simulink model "EKF_LQR_PID"  (R2024b)
settings: Solver=VariableStepAuto  StartTime=0.0  StopTime=10  FixedStep=0.001  RelTol=1e-3
values from neighbouring files (symbols this model uses):
  A = [0 1 0 0 0 0 ... (first row only)    [main.m]
  B = [0;1/mc;0;-1/mb;0;-1/(l*mc)]    [main.m]
  C = [1 0 0 0 l 0]    [main.m]
  dT = param.Ts    [main.m]
  Kd = 0.8    [main.m]
  Ki = 10    [main.m]
  Kp = 12    [main.m]
  l = 0.25    [main.m]
  L_gain = lqr(A,B,Q_LQR,R_LQR)    [main.m]
  LD = acker(system_l.A',system_l.C',poles)    [main.m]
  system_l = ss(A,B,C,D)    [main.m]
undefined symbols (not defined in the file or in its folder): denum, num, param
libraries: simulink x6, simulink_extras x6, slpidlib x1
settings Model: Creator=hospm  LastModifiedBy=elias

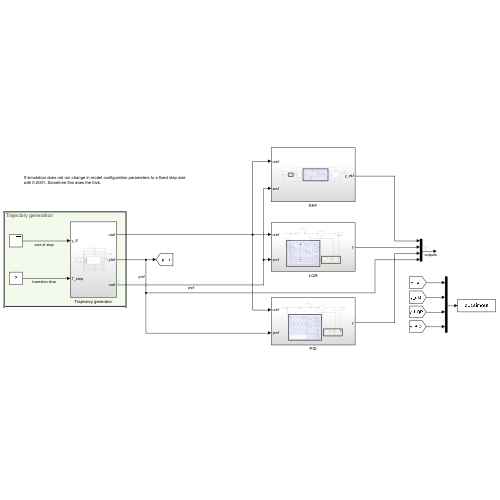
[thumbnail: Simulink's stored preview of the top-level diagram]
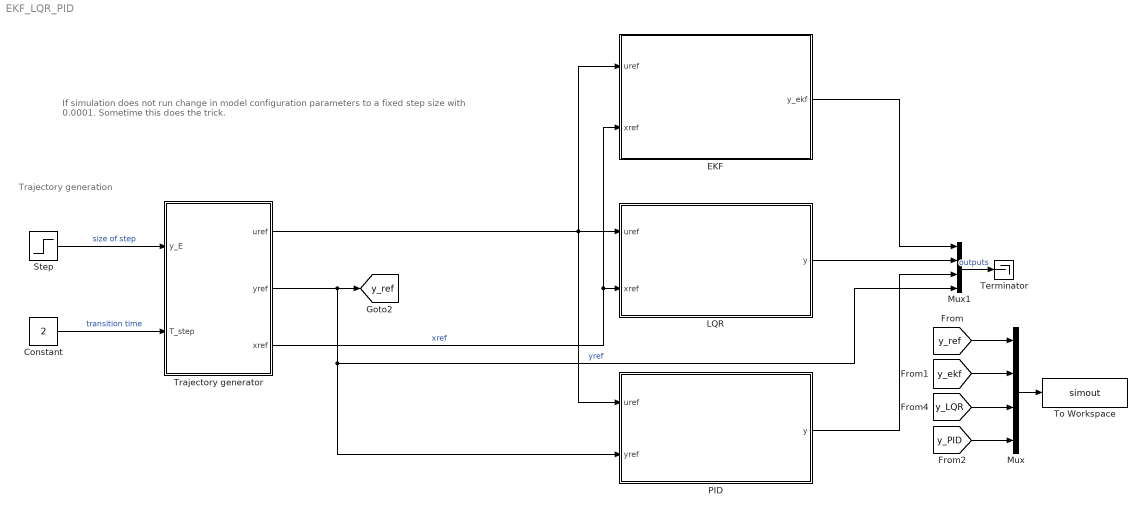
== system EKF_LQR_PID ==
  note: If simulation does not run change in model configuration parameters to a fixed step size with 0.0001. Sometime this does the trick.
  note: Trajectory generation
  Constant : Constant  Value=2
  EKF : Subsystem
  LQR : Subsystem
  Mux : Mux
  Mux1 : Mux
  PID : Subsystem
  Step : Step  Time=0  After=2  SampleTime=0
  Terminator : Terminator
  To Workspace : ToWorkspace  VariableName=simout  SaveFormat=Timeseries  SampleTime=-1
  Trajectory generator : Subsystem
  tag scope: y_ref=global
  wires:
  Constant/1 -> Trajectory generator/2(T_step)  "transition time"
  Trajectory generator/2(yref) -> Mux1/4, PID/2(yref), [y_ref]  "yref"
  Step/1 -> Trajectory generator/1(y_E)  "size of step"
  Mux/1 -> To Workspace/1
  [y_ref] -> Mux/1
  Trajectory generator/1(uref) -> PID/1(uref), EKF/1(uref), LQR/1(uref)
  Trajectory generator/3(xref) -> EKF/2(xref), LQR/2(xref)  "xref"
  EKF/1(y_ekf) -> Mux1/1
  Mux1/1 -> Terminator/1  "outputs"
  LQR/1(y) -> Mux1/2
  PID/1(y) -> Mux1/3
  [y_PID] -> Mux/4
  [y_LQR] -> Mux/3
  [y_ekf] -> Mux/2

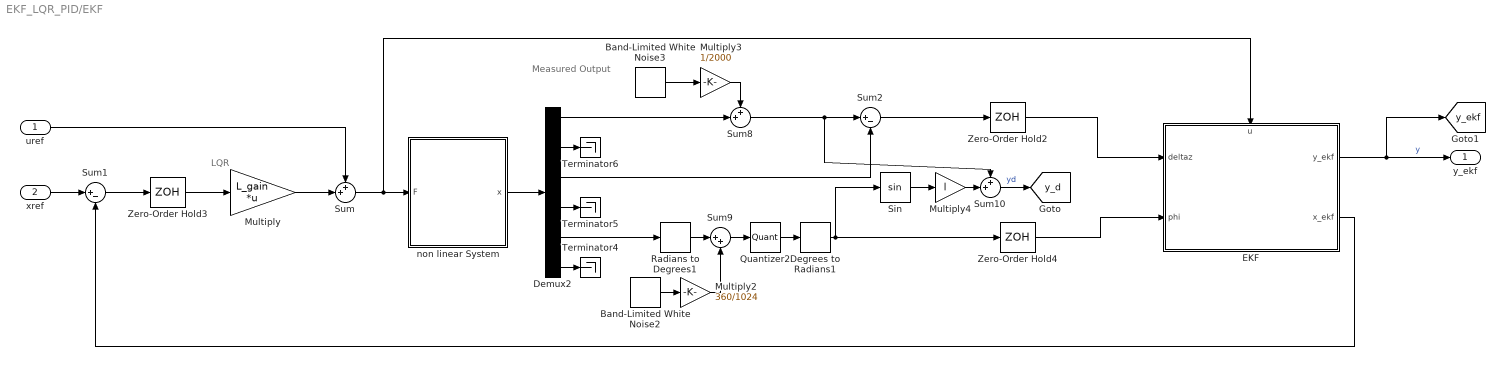
== system EKF_LQR_PID/EKF ==
  note: LQR
  note: Measured Output
  uref : Inport
  xref : Inport  Port=2
  Band-Limited White Noise2 : simulink/Sources/Band-Limited White Noise  Cov=[0.1]  Ts=0.1  seed=[23341]
  Band-Limited White Noise3 : simulink/Sources/Band-Limited White Noise  Cov=[0.1]  Ts=0.1  seed=[23341]
  Degrees to Radians1 : simulink_extras/Transformations/Degrees to Radians
  Demux2 : Demux  Outputs=6
  EKF : Subsystem
      settings: PortSchema="{\"entries\":[{\"content\":{\"sides\":[{\"content\":{\"connectorIds\":[\"In1\",\"In2\"]},\"type\":\"ConnectorPlacement.EquallySpacedRectSide\",\"uuid\":\"7d448900-18ad-41d5-8be7-5b2f8237e026\"},{\"content\":{\"connectorIds\":[\"Out1\",\"Out2\"],\"side\":\"RIGHT\"},\"type\":\"ConnectorPlacement.EquallySpacedRectSide\",\"uuid\":\"f5f89615-8db2-446f-9ddf-3fbf985b739e\"},{\"content\":{\"connectorIds\":[\"In3\"],\"side\":\"TOP\"},\"type\":\"ConnectorPlacement.EquallySpacedRectSide\",\"uuid\":\"59db8e0c-78e3-492a-b009-e31c80c69e55\"}]},\"type\":\"ConnectorPlacement.EquallySpacedConnector\",\"uuid\":\"488a84d0-998b-49ab-9f38-67f2321ad282\"}],\"packageUris\":[\"http://schema.mathworks.com/mf0/Connector/R2020b\"],\"version\":\"1.0\"}"
  Multiply : Gain  Gain=L_gain  Multiplication=Matrix(K*u) (u vector)
  Multiply2 : Gain  Gain=360/1024
  Multiply3 : Gain  Gain=1/2000
  Multiply4 : Gain  Gain=l
  Quantizer2 : Quantizer  QuantizationInterval=360/1024
  Radians to Degrees1 : simulink_extras/Transformations/Radians to Degrees
  Sin : Trigonometry
  Sum : Sum  Inputs=++|
  Sum1 : Sum  Inputs=|+-
  Sum10 : Sum  Inputs=++|
  Sum2 : Sum  Inputs=|+-
  Sum8 : Sum  Inputs=++|
  Sum9 : Sum  Inputs=|++
  Terminator4 : Terminator
  Terminator5 : Terminator
  Terminator6 : Terminator
  Zero-Order Hold2 : ZeroOrderHold  SampleTime=param.Ts
  Zero-Order Hold3 : ZeroOrderHold  SampleTime=param.Ts
  Zero-Order Hold4 : ZeroOrderHold  SampleTime=param.Ts
  non linear System : Subsystem
  y_ekf : Outport
  tag scope: y_d=global, y_ekf=global
  wires:
  Demux2/3 -> Sum2/2
  Multiply/1 -> Sum/2
  Degrees to Radians1/1 -> Sin/1, Zero-Order Hold4/1
  Sum9/1 -> Quantizer2/1
  Band-Limited White Noise3/1 -> Multiply3/1
  Zero-Order Hold3/1 -> Multiply/1
  EKF/2(x_ekf) -> Sum1/2
  Demux2/2 -> Terminator6/1
  Sum8/1 -> Sum2/1, Sum10/1
  Demux2/5 -> Radians to Degrees1/1
  Radians to Degrees1/1 -> Sum9/1
  Demux2/6 -> Terminator4/1
  Demux2/4 -> Terminator5/1
  Sum2/1 -> Zero-Order Hold2/1
  Multiply4/1 -> Sum10/2
  Multiply2/1 -> Sum9/2
  Multiply3/1 -> Sum8/1
  Sin/1 -> Multiply4/1
  Sum/1 -> EKF/3(u), non linear System/1(F)
  non linear System/1(x) -> Demux2/1
  uref/1 -> Sum/1
  Sum10/1 -> [y_d]  "yd"
  Quantizer2/1 -> Degrees to Radians1/1
  Zero-Order Hold2/1 -> EKF/1(deltaz)
  Band-Limited White Noise2/1 -> Multiply2/1
  Zero-Order Hold4/1 -> EKF/2(phi)
  Sum1/1 -> Zero-Order Hold3/1
  xref/1 -> Sum1/1
  Demux2/1 -> Sum8/2
  EKF/1(y_ekf) -> [y_ekf], y_ekf/1  "y"

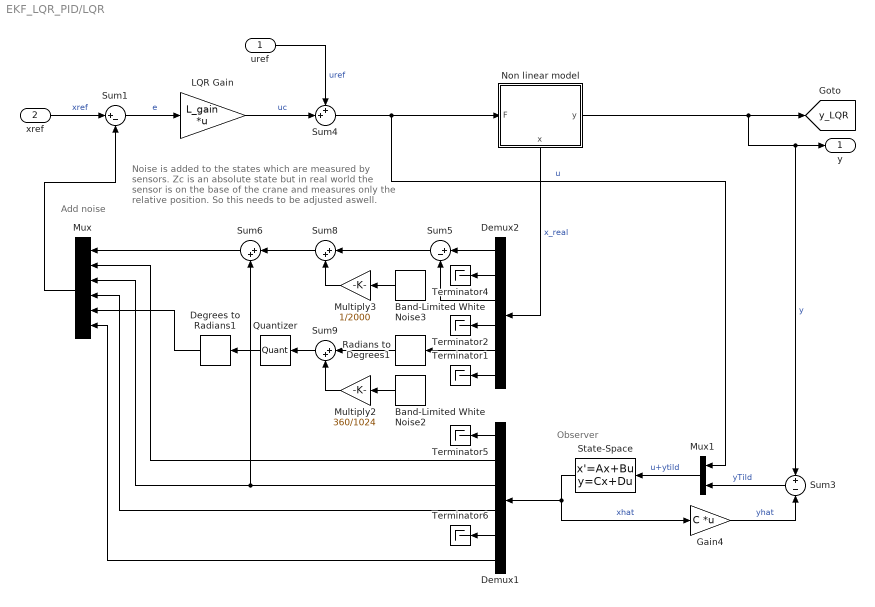
== system EKF_LQR_PID/LQR ==
  note: Add noise
  note: Noise is added to the states which are measured by sensors. Zc is an absolute state but in real world the sensor is on the base of the crane and measures only the relative position. So this needs to be adjusted aswell.
  note: Observer
  uref : Inport
  xref : Inport  Port=2
  Band-Limited White Noise2 : simulink/Sources/Band-Limited White Noise  Cov=[0.1]  Ts=0.1  seed=[23341]
  Band-Limited White Noise3 : simulink/Sources/Band-Limited White Noise  Cov=[0.1]  Ts=0.1  seed=[23341]
  Degrees to Radians1 : simulink_extras/Transformations/Degrees to Radians
  Demux1 : Demux  Outputs=6
  Demux2 : Demux  Outputs=6
  Gain4 : Gain  Gain=C  Multiplication=Matrix(K*u)
  LQR Gain : Gain  Gain=L_gain  Multiplication=Matrix(K*u) (u vector)
  Multiply2 : Gain  Gain=360/1024
  Multiply3 : Gain  Gain=1/2000
  Mux : Mux  Inputs=6
  Mux1 : Mux  Inputs=2
  Non linear model : Subsystem
      settings: PortSchema="{\"entries\":[{\"content\":{\"sides\":[{\"content\":{\"connectorIds\":[\"In1\"]},\"type\":\"ConnectorPlacement.EquallySpacedRectSide\",\"uuid\":\"1168ee74-8fd3-4705-8c7a-3655de58a2af\"},{\"content\":{\"connectorIds\":[\"Out1\"],\"side\":\"RIGHT\"},\"type\":\"ConnectorPlacement.EquallySpacedRectSide\",\"uuid\":\"a82eda53-f6cc-410c-ba8f-7e45612c6547\"},{\"content\":{\"side\":\"TOP\"},\"type\":\"ConnectorPlacement.EquallySpacedRectSide\",\"uuid\":\"a2319d43-b25c-4b1a-80d2-b40e879cc37d\"},{\"content\":{\"connectorIds\":[\"Out2\"],\"side\":\"BOTTOM\"},\"type\":\"ConnectorPlacement.EquallySpacedRectSide\",\"uuid\":\"4b95ead7-91aa-4544-96a9-9d2b2de2ef4c\"}]},\"type\":\"ConnectorPlacement.EquallySpacedConnector\",\"uuid\":\"35c66d5a-bdf4-4762-a518-3c02185c8911\"}],\"packageUris\":[\"http://schema.mathworks.com/mf0/Connector/R2020b\"],\"version\":\"1.0\"}"
  Quantizer : Quantizer  QuantizationInterval=360/1024
  Radians to Degrees1 : simulink_extras/Transformations/Radians to Degrees
  State-Space : StateSpace  A=system_l.A  B=[B LD']  C=eye(6)  D=zeros(6,2)  InitialCondition=0
  Sum1 : Sum  Inputs=|+-
  Sum3 : Sum  Inputs=+|-
  Sum4 : Sum  Inputs=++|
  Sum5 : Sum  Inputs=|+-
  Sum6 : Sum  Inputs=|++
  Sum8 : Sum  Inputs=|++
  Sum9 : Sum  Inputs=|++
  Terminator{1..2,4..6} (5 alike) : Terminator
  y : Outport
  tag scope: y_LQR=global
  wires:
  Sum4/1 -> Non linear model/1(F), Mux1/1  "u"
  Quantizer/1 -> Degrees to Radians1/1
  LQR Gain/1 -> Sum4/2  "uc"
  Demux2/6 -> Terminator1/1
  Demux2/5 -> Radians to Degrees1/1
  Multiply2/1 -> Sum9/2
  Band-Limited White Noise3/1 -> Multiply3/1
  Multiply3/1 -> Sum8/2
  Degrees to Radians1/1 -> Mux/5
  Demux2/1 -> Sum5/1
  xref/1 -> Sum1/1  "xref"
  Sum1/1 -> LQR Gain/1  "e"
  Mux/1 -> Sum1/2
  Radians to Degrees1/1 -> Sum9/1
  uref/1 -> Sum4/1  "uref"
  Demux2/2 -> Terminator4/1
  Band-Limited White Noise2/1 -> Multiply2/1
  Demux2/4 -> Terminator2/1
  Sum9/1 -> Quantizer/1
  Demux2/3 -> Sum5/2
  Non linear model/1(y) -> [y_LQR], y/1, Sum3/1  "y"
  Mux1/1 -> State-Space/1  "u+ytild"
  Gain4/1 -> Sum3/2  "yhat"
  State-Space/1 -> Demux1/1, Gain4/1  "xhat"
  Sum3/1 -> Mux1/2  "yTild"
  Non linear model/2(x) -> Demux2/1  "x_real"
  Demux1/1 -> Terminator5/1
  Demux1/5 -> Terminator6/1
  Demux1/6 -> Mux/6
  Demux1/4 -> Mux/4
  Demux1/3 -> Mux/3, Sum6/2
  Demux1/2 -> Mux/2
  Sum5/1 -> Sum8/1
  Sum8/1 -> Sum6/1
  Sum6/1 -> Mux/1

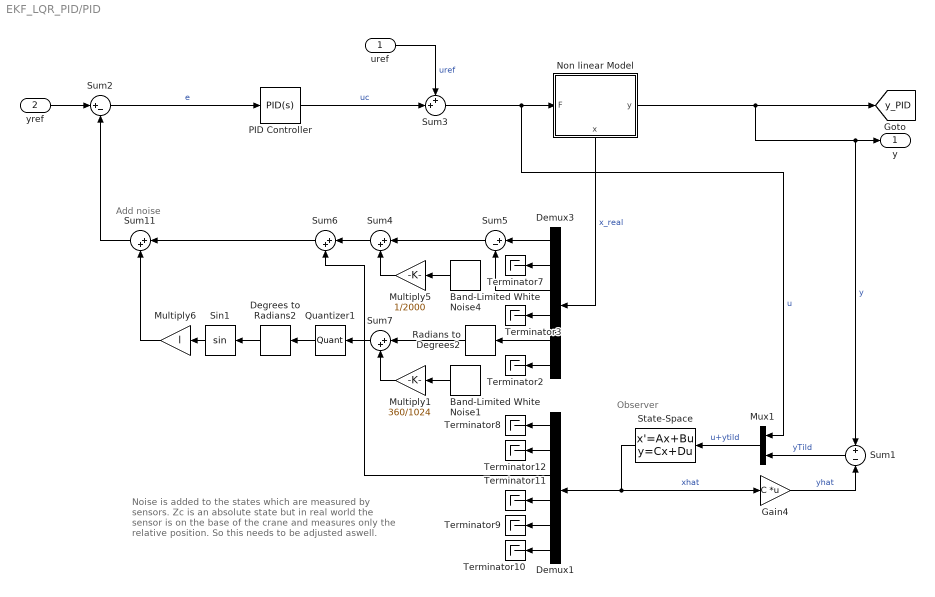
== system EKF_LQR_PID/PID ==
  note: Observer
  note: Add noise
  note: Noise is added to the states which are measured by sensors. Zc is an absolute state but in real world the sensor is on the base of the crane and measures only the relative position. So this needs to be adjusted aswell.
  uref : Inport
  yref : Inport  Port=2
  Band-Limited White Noise1 : simulink/Sources/Band-Limited White Noise  Cov=[0.1]  Ts=0.1  seed=[23341]
  Band-Limited White Noise4 : simulink/Sources/Band-Limited White Noise  Cov=[0.1]  Ts=0.1  seed=[23341]
  Degrees to Radians2 : simulink_extras/Transformations/Degrees to Radians
  Demux1 : Demux  Outputs=6
  Demux3 : Demux  Outputs=6
  Gain4 : Gain  Gain=C  Multiplication=Matrix(K*u)
  Multiply1 : Gain  Gain=360/1024
  Multiply5 : Gain  Gain=1/2000
  Multiply6 : Gain  Gain=l
  Mux1 : Mux  Inputs=2
  Non linear Model : Subsystem
      settings: PortSchema="{\"entries\":[{\"content\":{\"sides\":[{\"content\":{\"connectorIds\":[\"In1\"]},\"type\":\"ConnectorPlacement.EquallySpacedRectSide\",\"uuid\":\"1168ee74-8fd3-4705-8c7a-3655de58a2af\"},{\"content\":{\"connectorIds\":[\"Out1\"],\"side\":\"RIGHT\"},\"type\":\"ConnectorPlacement.EquallySpacedRectSide\",\"uuid\":\"a82eda53-f6cc-410c-ba8f-7e45612c6547\"},{\"content\":{\"side\":\"TOP\"},\"type\":\"ConnectorPlacement.EquallySpacedRectSide\",\"uuid\":\"a2319d43-b25c-4b1a-80d2-b40e879cc37d\"},{\"content\":{\"connectorIds\":[\"Out2\"],\"side\":\"BOTTOM\"},\"type\":\"ConnectorPlacement.EquallySpacedRectSide\",\"uuid\":\"4b95ead7-91aa-4544-96a9-9d2b2de2ef4c\"}]},\"type\":\"ConnectorPlacement.EquallySpacedConnector\",\"uuid\":\"35c66d5a-bdf4-4762-a518-3c02185c8911\"}],\"packageUris\":[\"http://schema.mathworks.com/mf0/Connector/R2020b\"],\"version\":\"1.0\"}"
  PID Controller : slpidlib/PID Controller  Controller=PID  Form=Parallel  TimeDomain=Continuous-time  UseExternalTs=off  SampleTime=-1  IntegratorMethod=Forward Euler  FilterMethod=Forward Euler  ControllerParametersSource=internal  P=Kp  I=Ki  UseKiTs=off  D=Kd  UseExternalDerivativeSource=off  N=100  UseFilter=on  TunerSelectOption=Transfer Function Based (PID Tuner App)  InitialConditionSource=internal  InitialConditionForIntegrator=0  InitialConditionForFilter=0  DifferentiatorICPrevScaledInput=0  ExternalReset=none  TrackingMode=off  Kt=1  LimitOutput=off  SatLimitsSource=internal  UpperSaturationLimit=inf  LowerSaturationLimit=-inf  LinearizeAsGain=on  AntiWindupMode=none  Kb=1  LimitIntegrator=off  UpperIntegratorSaturationLimit=inf  LowerIntegratorSaturationLimit=-inf  POutMin=[]  POutMax=[]  IOutMin=[]  IOutMax=[]  DOutMin=[]  DOutMax=[]  NOutMin=[]  NOutMax=[]  SumOutMin=[]  SumOutMax=[]  SaturationOutMin=[]  SaturationOutMax=[]  PParamMin=[]  PParamMax=[]  IParamMin=[]  IParamMax=[]  DParamMin=[]  DParamMax=[]  NParamMin=[]  NParamMax=[]  KbParamMin=[]  KbParamMax=[]  KtParamMin=[]  KtParamMax=[]  KbOutMin=[]  KbOutMax=[]  KtOutMin=[]  KtOutMax=[]  IntegratorOutMin=[]  IntegratorOutMax=[]  FilterOutMin=[]  FilterOutMax=[]  SumI1OutMin=[]  SumI1OutMax=[]  SumI2OutMin=[]  SumI2OutMax=[]  SumI3OutMin=[]  SumI3OutMax=[]  SumI4OutMin=[]  SumI4OutMax=[]  SumDOutMin=[]  SumDOutMax=[]  DifferentiatorOutMin=[]  DifferentiatorOutMax=[]  FilterDiffOutCoefMin=[]  FilterDiffOutCoefMax=[]  ReciprocalOutMin=[]  ReciprocalOutMax=[]  SumDenOutMin=[]  SumDenOutMax=[]  SumNumOutMin=[]  SumNumOutMax=[]  DivideOutMin=[]  DivideOutMax=[]  UdiffTsProdOutMin=[]  UdiffTsProdOutMax=[]  NTsProdOutMin=[]  NTsProdOutMax=[]  UintegralTsProdOutMin=[]  UintegralTsProdOutMax=[]  UngainTsProdOutMin=[]  UngainTsProdOutMax=[]  ClampingZeroOutDataTypeStr=Inherit: Inherit via back propagation  ClampingZeroOutMin=[]  ClampingZeroOutMax=[]  FilterDenConstantOutDataTypeStr=Inherit: Inherit via back propagation  FilterDenConstantOutMin=[]  FilterDenConstantOutMax=[]  PCopyOutDataTypeStr=Inherit: Inherit via back propagation  PCopyOutMin=[]  PCopyOutMax=[]  NCopyOutDataTypeStr=Inherit: Inherit via back propagation  NCopyOutMin=[]  NCopyOutMax=[]  IntegratorContinuousStateAttributes=''  IntegratorStateMustResolveToSignalObject=off  IntegratorRTWStateStorageClass=Auto  FilterContinuousStateAttributes=''  FilterStateMustResolveToSignalObject=off  FilterRTWStateStorageClass=Auto  ParallelPVariant=InternalParameters  IdealPVariant=Disabled  IVariant=InternalParameters  DVariant=InternalParameters  IntegratorVariant=Continuous  SatVariant=Disabled  AWVariant=Passthrough  PCopyVariant=Disabled  TRVariant=Disabled  FdbkBlocksVariant=Forward  IdealPFdbkVariant=Disabled  SatFdbkVariant=Disabled  DerivativeFilterVariant=ContFilter  NVariant=InternalParameters  NCopyVariant=Disabled  FilterICVariant=InternalICsFilter  IntegratorICVariant=InternalICs  ExternalResetVariant=Disabled  TRSumVariant=Passthrough  SumFdbkVariant=Disabled  SumVariant=Sum_PID  TsampFilterVariant=InternalTs  TsampNgainVariant=Passthrough  TsampIntegralVariant=Disabled_SignalSpec  ExternalSaturationOutDataTypeStr=Inherit: Same as second input  DerivativeSourceVariant=ErrorSignal  PreIntVariant=InternalPreInt
  Quantizer1 : Quantizer  QuantizationInterval=360/1024
  Radians to Degrees2 : simulink_extras/Transformations/Radians to Degrees
  Sin1 : Trigonometry
  State-Space : StateSpace  A=system_l.A  B=[B LD']  C=eye(6)  D=zeros(6,2)  InitialCondition=0
  Sum1 : Sum  Inputs=+|-
  Sum{4,6..7,11} (4 alike) : Sum  Inputs=|++
  Sum2 : Sum  Inputs=|+-
  Sum3 : Sum  Inputs=++|
  Sum5 : Sum  Inputs=|+-
  Terminator{2..3,7..12} (8 alike) : Terminator
  y : Outport
  tag scope: y_PID=global
  wires:
  Sum2/1 -> PID Controller/1  "e"
  PID Controller/1 -> Sum3/2  "uc"
  uref/1 -> Sum3/1  "uref"
  Sum3/1 -> Non linear Model/1(F), Mux1/1  "u"
  yref/1 -> Sum2/1
  Sum1/1 -> Mux1/2  "yTild"
  Gain4/1 -> Sum1/2  "yhat"
  Non linear Model/1(y) -> y/1, Sum1/1, [y_PID]  "y"
  Mux1/1 -> State-Space/1  "u+ytild"
  Sum5/1 -> Sum4/1
  Demux3/1 -> Sum5/1
  Demux1/5 -> Terminator9/1
  Demux3/4 -> Terminator3/1
  Demux1/3 -> Sum6/2
  Radians to Degrees2/1 -> Sum7/1
  Multiply1/1 -> Sum7/2
  Demux1/6 -> Terminator10/1
  Multiply5/1 -> Sum4/2
  Demux3/5 -> Radians to Degrees2/1
  Band-Limited White Noise4/1 -> Multiply5/1
  Non linear Model/2(x) -> Demux3/1  "x_real"
  Demux1/1 -> Terminator8/1
  Band-Limited White Noise1/1 -> Multiply1/1
  Demux1/4 -> Terminator11/1
  State-Space/1 -> Demux1/1, Gain4/1  "xhat"
  Degrees to Radians2/1 -> Sin1/1
  Sum4/1 -> Sum6/1
  Demux3/2 -> Terminator7/1
  Demux1/2 -> Terminator12/1
  Sum11/1 -> Sum2/2
  Sum7/1 -> Quantizer1/1
  Demux3/3 -> Sum5/2
  Quantizer1/1 -> Degrees to Radians2/1
  Sum6/1 -> Sum11/1
  Demux3/6 -> Terminator2/1
  Multiply6/1 -> Sum11/2
  Sin1/1 -> Multiply6/1

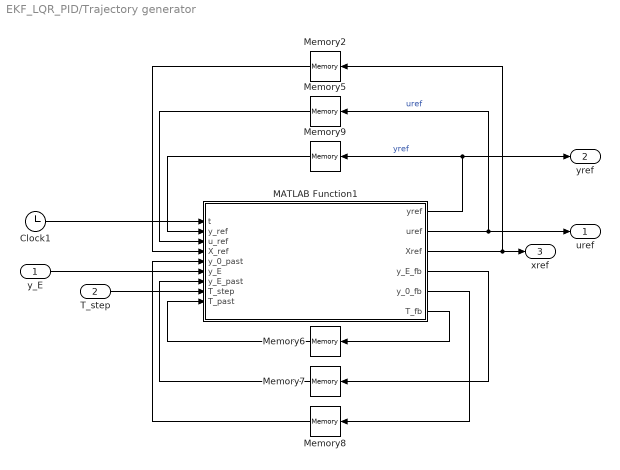
== system EKF_LQR_PID/Trajectory generator ==
  y_E : Inport
  T_step : Inport  Port=2
  Clock1 : Clock
  MATLAB Function1 : MATLAB Function  TreatAsAtomicUnit=on
  Memory2 : Memory  InitialCondition=zeros(6,1)
  Memory{5..9} (5 alike) : Memory
  uref : Outport
  yref : Outport  Port=2
  xref : Outport  Port=3
  wires:
  Clock1/1 -> MATLAB Function1/1(t)
  Memory7/1 -> MATLAB Function1/7(y_E_past)
  MATLAB Function1/6(T_fb) -> Memory6/1
  Memory6/1 -> MATLAB Function1/9(T_past)
  MATLAB Function1/1(yref) -> yref/1, Memory9/1  "yref"
  Memory9/1 -> MATLAB Function1/2(y_ref)
  Memory5/1 -> MATLAB Function1/3(u_ref)
  Memory8/1 -> MATLAB Function1/5(y_0_past)
  MATLAB Function1/5(y_0_fb) -> Memory8/1
  MATLAB Function1/4(y_E_fb) -> Memory7/1
  y_E/1 -> MATLAB Function1/6(y_E)
  T_step/1 -> MATLAB Function1/8(T_step)
  MATLAB Function1/2(uref) -> uref/1, Memory5/1  "uref"
  MATLAB Function1/3(Xref) -> Memory2/1, xref/1
  Memory2/1 -> MATLAB Function1/4(X_ref)

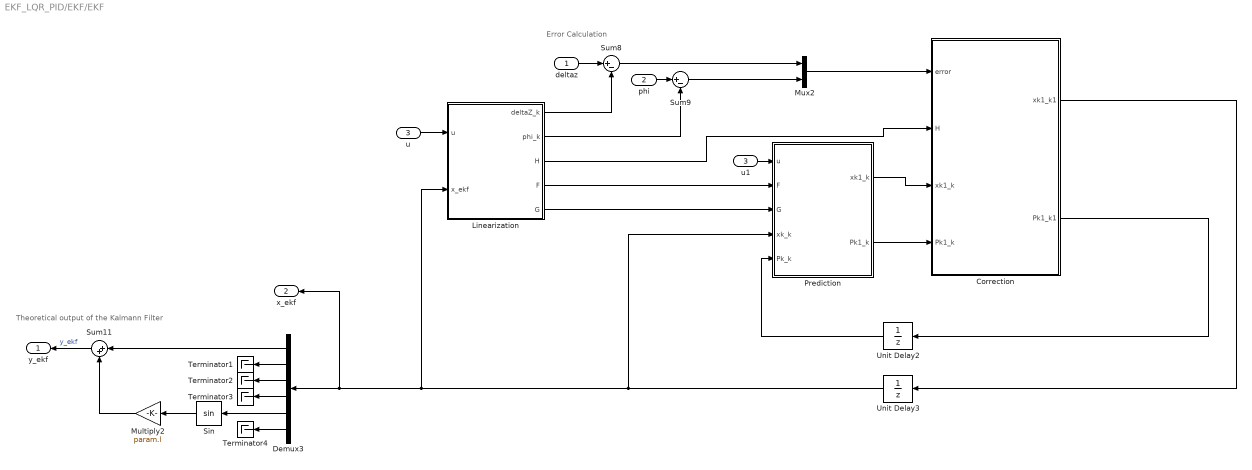
== system EKF_LQR_PID/EKF/EKF ==
  note: Theoretical output of the Kalmann Filter
  note: Error Calculation
  deltaz : Inport
  phi : Inport  Port=2
  u : Inport  Port=3
  Correction : MATLAB Function  TreatAsAtomicUnit=on
  Demux3 : Demux  Outputs=6
  Linearization : MATLAB Function  TreatAsAtomicUnit=on
  Multiply2 : Gain  Gain=param.l
  Mux2 : Mux  Inputs=2
  Prediction : MATLAB Function  TreatAsAtomicUnit=on
  Sin : Trigonometry
  Sum11 : Sum  Inputs=|++
  Sum8 : Sum  Inputs=|+-
  Sum9 : Sum  Inputs=|+-
  Terminator{1..4} (4 alike) : Terminator
  Unit Delay2 : UnitDelay  SampleTime=param.Ts  HasFrameUpgradeWarning=on
  Unit Delay3 : UnitDelay  InitialCondition=[0 0 0 0 0 0]'  SampleTime=param.Ts  HasFrameUpgradeWarning=on
  u1 : InportShadow  Port=3
  y_ekf : Outport
  x_ekf : Outport  Port=2
  wires:
  Unit Delay2/1 -> Prediction/5(Pk_k)
  Linearization/4(F) -> Prediction/2(F)
  Multiply2/1 -> Sum11/2
  Mux2/1 -> Correction/1(error)
  Prediction/1(xk1_k) -> Correction/3(xk1_k)
  Sin/1 -> Multiply2/1
  Linearization/1(deltaZ_k) -> Sum8/2
  u/1 -> Linearization/1(u)
  Correction/2(Pk1_k1) -> Unit Delay2/1
  Linearization/2(phi_k) -> Sum9/2
  Unit Delay3/1 -> Prediction/4(xk_k), Linearization/2(x_ekf), x_ekf/1, Demux3/1
  Linearization/3(H) -> Correction/2(H)
  Correction/1(xk1_k1) -> Unit Delay3/1
  Linearization/5(G) -> Prediction/3(G)
  Sum8/1 -> Mux2/1
  Sum9/1 -> Mux2/2
  Prediction/2(Pk1_k) -> Correction/4(Pk1_k)
  Sum11/1 -> y_ekf/1  "y_ekf"
  Demux3/1 -> Sum11/1
  Demux3/5 -> Sin/1
  deltaz/1 -> Sum8/1
  phi/1 -> Sum9/1
  u1/1 -> Prediction/1(u)
  Demux3/2 -> Terminator1/1
  Demux3/4 -> Terminator3/1
  Demux3/6 -> Terminator4/1
  Demux3/3 -> Terminator2/1

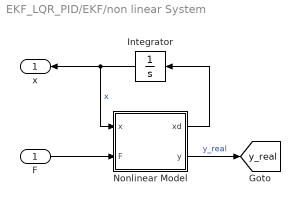
== system EKF_LQR_PID/EKF/non linear System ==
  F : Inport
  Integrator : Integrator  InitialCondition=[0;0;0;0;0;0]
  Nonlinear Model : MATLAB Function  TreatAsAtomicUnit=on
  x : Outport
  tag scope: y_real=global
  wires:
  F/1 -> Nonlinear Model/2(F)
  Integrator/1 -> Nonlinear Model/1(x), x/1  "x"
  Nonlinear Model/1(xd) -> Integrator/1
  Nonlinear Model/2(y) -> [y_real]  "y_real"

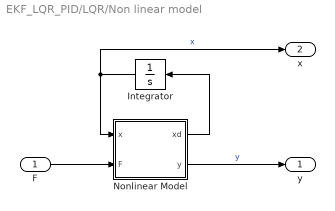
== system EKF_LQR_PID/LQR/Non linear model ==
  F : Inport
  Integrator : Integrator  InitialCondition=[0;0;0;0;0;0]
  Nonlinear Model : MATLAB Function  TreatAsAtomicUnit=on
  y : Outport
  x : Outport  Port=2
  wires:
  F/1 -> Nonlinear Model/2(F)
  Integrator/1 -> Nonlinear Model/1(x), x/1  "x"
  Nonlinear Model/2(y) -> y/1  "y"
  Nonlinear Model/1(xd) -> Integrator/1

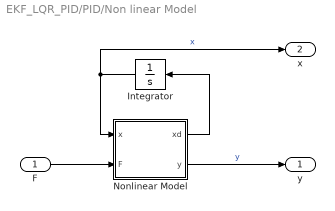
== system EKF_LQR_PID/PID/Non linear Model ==
  F : Inport
  Integrator : Integrator  InitialCondition=[0;0;0;0;0;0]
  Nonlinear Model : MATLAB Function  TreatAsAtomicUnit=on
  y : Outport
  x : Outport  Port=2
  wires:
  Nonlinear Model/1(xd) -> Integrator/1
  Nonlinear Model/2(y) -> y/1  "y"
  Integrator/1 -> x/1, Nonlinear Model/1(x)  "x"
  F/1 -> Nonlinear Model/2(F)

== matlab function EKF_LQR_PID/EKF/EKF/Prediction ==
  data: u input; xk1_k output; F input; Pk1_k output; G input; xk_k input; Pk_k input; param parameter
function [xk1_k, Pk1_k] = prediction(u, F, G, xk_k, Pk_k, param)
Q = param.Q;

xk1_k = F*xk_k+G*u;


Pk1_k = F*Pk_k*F'+Q;

== matlab function EKF_LQR_PID/EKF/EKF/Linearization ==
  data: deltaZ_k output; u input; phi_k output; H output; x_ekf input; F output; G output; param parameter
function [deltaZ_k, phi_k, H, F, G] = jacob(u, x_ekf,param)

    %get parameters from param
    mb = param.mb;
    mc = param.mc;
    ml = param.ml;
    
    kb = param.kb;
    kc = param.kc;
    
    db = param.db;
    dc = param.dc;
    
    l  = param.l;
    g  = param.g;
    Ts= param.Ts;
    
    %reconstruction states
    Zc = x_ekf(1);
    dZc = x_ekf(2);
    Zb = x_ekf(3);
    dZb = x_ekf(4);
    Phi = x_ekf(5);
    dPhi = x_ekf(6);

    % Jacobians
    B_jacob=[0;
            1/(- ml*cos(Phi)^2 + mc + ml);
                                        0;
                                    -1/mb;
                                        0;
            -cos(Phi)/(l*(- ml*cos(Phi)^2 + mc + ml))];

    A_jacob=[0,1,0,0,0,0;
                0,-dc/(- ml*cos(Phi)^2 + mc + ml),0,...
                dc/(- ml*cos(Phi)^2 + mc + ml),...
                (l*ml*dPhi^2*cos(Phi) + g*ml*cos(Phi)^2 - g*ml*sin(Phi)^2)/(- ml*cos(Phi)^2 + mc + ml) - (2*ml*cos(Phi)*sin(Phi)*(l*ml*sin(Phi)*dPhi^2 + u + dZb*dc - dZc*dc + g*ml*cos(Phi)*sin(Phi)))/(- ml*cos(Phi)^2 + mc + ml)^2,...
                (2*dPhi*l*ml*sin(Phi))/(- ml*cos(Phi)^2 + mc + ml);
                0,0,0,1,0,0;
                0,dc/mb, -kb/mb,-(db + dc)/mb,0,0;
                0,0,0,0,0,1;
                0, (dc*cos(Phi))/(l*(- ml*cos(Phi)^2 + mc + ml)),0,...
                -(dc*cos(Phi))/(l*(- ml*cos(Phi)^2 + mc + ml)),...
                (2*ml*cos(Phi)*sin(Phi)*(l*ml*cos(Phi)*sin(Phi)*dPhi^2 + u*cos(Phi) + dZb*dc*cos(Phi) - dZc*dc*cos(Phi) + g*mc*sin(Phi) + g*ml*sin(Phi)))/(l*(- ml*cos(Phi)^2 + mc + ml)^2) - (g*mc*cos(Phi) - u*sin(Phi) + g*ml*cos(Phi) - dZb*dc*sin(Phi) + dZc*dc*sin(Phi) + dPhi^2*l*ml*cos(Phi)^2 - dPhi^2*l*ml*sin(Phi)^2)/(l*(- ml*cos(Phi)^2 + mc + ml)),...
                -(2*dPhi*ml*cos(Phi)*sin(Phi))/(- ml*cos(Phi)^2 + mc + ml)];

    C_jacob=[1, 0, -1, 0, 0, 0;
            0, 0, 0, 0, 1, 0];




   phi_k = x_ekf(5);
   deltaZ_k = x_ekf(1)-x_ekf(3);
   F = eye(6)+A_jacob*Ts;
   G = B_jacob*Ts;
   H = C_jacob; %assume that C_jacob is time discret

== matlab function EKF_LQR_PID/EKF/EKF/Correction ==
  data: error input; xk1_k1 output; H input; xk1_k input; Pk1_k input; Pk1_k1 output; param parameter
function [xk1_k1, Pk1_k1] = correction(error, H, xk1_k, Pk1_k, param)
    Q = param.Q;
    R = param.R;

    K = Pk1_k*H'/(H*Pk1_k*H'+R);

    xk1_k1 = xk1_k+K*(error);

    Pk1_k1 = (eye(6)-K*H)*Pk1_k;

== matlab function EKF_LQR_PID/EKF/non linear System/Nonlinear Model ==
  data: x input; xd output; F input; param parameter; y output
function [xd, y]   = fcn(x,F,param)
% get variables
dc=param.dc;
db_real=param.db_real;
kb=param.kb;
l=param.l;
ml=param.ml;
mc=param.mc;
mb_real=param.mb_real;
g=param.g;

%This is the non linear state space modell
xd=zeros(6,1);
%get states from x
zc=x(1);
zcd=x(2);
zb=x(3);
zbd=x(4);
phi=x(5);
phid=x(6);

%Line for zcd
xd(1)=zcd;
%line for zcdd
xd(2)=(-zcd*dc+zbd*dc+phid^2*l*ml*sin(phi)+F+g*ml*cos(phi)*sin(phi))...
   /(-ml*cos(phi)^2+mc+ml);
%line for zbd
xd(3)=zbd;
%line for zbdd
xd(4)=-((-zcd*dc+zb*kb+zbd*(db_real+dc)+F)/mb_real);
%line for phid
xd(5)=phid;
%line for phidd
xd(6)=-((-zcd*dc*cos(phi)+zbd*dc*cos(phi)+phid^2*l*ml*cos(phi)*sin(phi)...
    +F*cos(phi)+g*sin(phi)*(mc+ml))/(l*(-ml*cos(phi)^2+mc+ml)));

y=zc+l*sin(phi);

== matlab function EKF_LQR_PID/PID/Non linear Model/Nonlinear Model ==
  data: x input; xd output; F input; y output; param parameter
function [xd, y]   = fcn(x,F,param)
% get variables
dc=param.dc;
db_real=param.db_real;
kb=param.kb;
l=param.l;
ml=param.ml;
mc=param.mc;
mb_real=param.mb_real;
g=param.g;

%This is the non linear state space modell
xd=zeros(6,1);
%get states from x
zc=x(1);
zcd=x(2);
zb=x(3);
zbd=x(4);
phi=x(5);
phid=x(6);

%Line for zcd
xd(1)=zcd;
%line for zcdd
xd(2)=(-zcd*dc+zbd*dc+phid^2*l*ml*sin(phi)+F+g*ml*cos(phi)*sin(phi))...
   /(-ml*cos(phi)^2+mc+ml);
%line for zbd
xd(3)=zbd;
%line for zbdd
xd(4)=-((-zcd*dc+zb*kb+zbd*(db_real+dc)+F)/mb_real);
%line for phid
xd(5)=phid;
%line for phidd
xd(6)=-((-zcd*dc*cos(phi)+zbd*dc*cos(phi)+phid^2*l*ml*cos(phi)*sin(phi)...
    +F*cos(phi)+g*sin(phi)*(mc+ml))/(l*(-ml*cos(phi)^2+mc+ml)));

y=zc+l*sin(phi);

== matlab function EKF_LQR_PID/LQR/Non linear model/Nonlinear Model ==
  data: x input; xd output; F input; y output; param parameter
function [xd, y]   = fcn(x,F,param)
% get variables
dc=param.dc;
db_real=param.db_real;
kb=param.kb;
l=param.l;
ml=param.ml;
mc=param.mc;
mb_real=param.mb_real;
g=param.g;

%This is the non linear state space modell
xd=zeros(6,1);
%get states from x
zc=x(1);
zcd=x(2);
zb=x(3);
zbd=x(4);
phi=x(5);
phid=x(6);

%Line for zcd
xd(1)=zcd;
%line for zcdd
xd(2)=(-zcd*dc+zbd*dc+phid^2*l*ml*sin(phi)+F+g*ml*cos(phi)*sin(phi))...
   /(-ml*cos(phi)^2+mc+ml);
%line for zbd
xd(3)=zbd;
%line for zbdd
xd(4)=-((-zcd*dc+zb*kb+zbd*(db_real+dc)+F)/mb_real);
%line for phid
xd(5)=phid;
%line for phidd
xd(6)=-((-zcd*dc*cos(phi)+zbd*dc*cos(phi)+phid^2*l*ml*cos(phi)*sin(phi)...
    +F*cos(phi)+g*sin(phi)*(mc+ml))/(l*(-ml*cos(phi)^2+mc+ml)));

y=zc+l*sin(phi);

== matlab function EKF_LQR_PID/Trajectory generator/MATLAB Function1 ==
  data: yref output; uref output; Xref output; t input; y_ref input; u_ref input; X_ref input; y_0_past input; y_E input; y_E_past input; T_step input; T_past input; num parameter; denum parameter; y_E_fb output; y_0_fb output; T_fb output; dT parameter; A parameter; B parameter
function [yref, uref, Xref, y_E_fb, y_0_fb, T_fb] = trajectory_planning(t, y_ref, u_ref, X_ref, y_0_past, y_E, y_E_past, T_step, T_past,num, denum, dT, A, B)
    % t: Current simulation time
    % y_0: Initial position
    % y_T: Desired position
    % T: Duration of the trajectory
    % num: Numerator of the Transferfunction
    % denum: Denumerator of the Transferfunction
    % n: Order of the system
    n=6;
    if(y_E==y_E_past) % still in the same transition
        y_0=y_0_past;
    else    % start of new transition
        y_0=y_ref;
        T_past=t;
    end
    
     % Normalize the current time
    tau=(t-T_past)/T_step;
 
    if(t<T_past+T_step)
        % Initialize coefficient matrix
        phi=zeros(n+1,2*n+2);
    
        % Fill the first row of the coefficient matrix
        for k=0:n
        phi(1,n+1-k)=nchoosek(n,k)*(-1)^k/(n+k+1);
        end
        
        % Add factor (which is multiplied by the sum) to all coefficients
        phi=factorial(2*n+1)/factorial(n)^2*phi;
        
        for j=1:n
        phi(j+1,j+1:end)=1/T_step*polyder(phi(j,j:end));
        end
        
        phi4=zeros(n+1,length(tau));
        
        for i=1:n+1
            phi4(i,:)=polyval(phi(i,:),tau);
        end
        
        % Compute the scaled trajectory
        b0=num(end); % Scaling factor is equal to b0 of numerator polynomial
        yf=1/b0*(y_E-y_0)*phi4; % add the scaling factor to the prototype-function
        yf(1,:)=y_0/b0+yf(1,:);

        YF=flipud(yf);
    
        uref=denum*YF;
        yref=num*YF;
        Xref = X_ref + dT * (A * X_ref + B * uref);
    else
        uref=u_ref;
        yref=y_ref;
        Xref = X_ref;
    end
    T_fb=T_past;
    y_0_fb=y_0;
    y_E_fb=y_E;
    
end
